simulink model "RobotRuka2012B"  (R2012b)
settings: Solver=ode45  SolverMode=SingleTasking  StartTime=0.0  StopTime=10.0  RelTol=1e-3
undefined symbols (not defined in the file): g, Kd, Kp, lc1, m0, m1, m2
libraries: fuzblock x2
settings Model: CovMetricSettings=dwe  CovHtmlReporting=off  covSaveCumulativeToWorkspaceVar=off  CovSaveSingleToWorkspaceVar=off  CovExternalEMLEnable=on  Creator=Aldin  LastModifiedBy=Aldin
settings DataIOCC: LimitDataPoints=off  SaveFormat=StructureWithTime  ReturnWorkspaceOutputs=on
settings OptimizationCC: ExpressionDepthLimit=128
settings DebuggingCC: UnderspecifiedInitializationDetection=Simplified  MergeDetectMultiDrivingBlocksExec=error  SolverPrmCheckMsg=none  FrameProcessingCompatibilityMsg=error  StateNameClashWarn=none  SFUnexpectedBacktrackingDiag=error  SFNoUnconditionalDefaultTransitionDiag=error
settings HardwareCC: ProdBitPerPointer=64  ProdLargestAtomicFloat=Float  ProdIntDivRoundTo=Zero  ProdEndianess=LittleEndian  ProdHWDeviceType=Specified
settings ModelReferenceCC: PropagateSignalLabelsOutOfModel=on
settings SFSimCC: SimUseLocalCustomCode=on
settings RTWCC: RTWUseLocalCustomCode=on
settings CodeAppCC: CustomSymbolStrType=$N$R$M_T
settings GRTTargetCC: CodeReplacementLibrary=C99 (ISO)

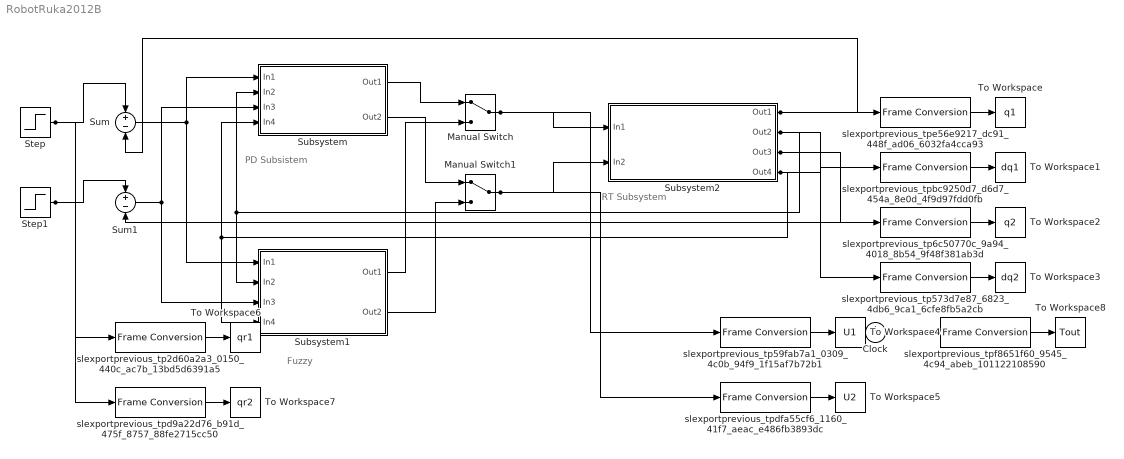
== system RobotRuka2012B ==
  note: PD Subsistem
  note: Fuzzy
  note: RT Subsystem
  Clock : Clock
  Manual Switch : ManualSwitch
  Manual Switch1 : ManualSwitch
  Step : Step  Time=0  SampleTime=0
  Step1 : Step  Time=0  SampleTime=0
  Subsystem : Subsystem
  Subsystem1 : Subsystem
  Subsystem2 : Subsystem
  Sum : Sum  Inputs=+-
  Sum1 : Sum  Inputs=+-
  To Workspace : ToWorkspace  VariableName=q1  SampleTime=-1
  To Workspace1 : ToWorkspace  VariableName=dq1  SampleTime=-1
  To Workspace2 : ToWorkspace  VariableName=q2  SampleTime=-1
  To Workspace3 : ToWorkspace  VariableName=dq2  SampleTime=-1
  To Workspace4 : ToWorkspace  VariableName=U1  SampleTime=-1
  To Workspace5 : ToWorkspace  VariableName=U2  SampleTime=-1
  To Workspace6 : ToWorkspace  VariableName=qr1  SampleTime=-1
  To Workspace7 : ToWorkspace  VariableName=qr2  SampleTime=-1
  To Workspace8 : ToWorkspace  VariableName=Tout  SampleTime=-1
  slexportprevious_tp2d60a2a3_0150_440c_ac7b_13bd5d6391a5 : FrameConversion  OutFrame=Sample-based
  slexportprevious_tp573d7e87_6823_4db6_9ca1_6cfe8fb5a2cb : FrameConversion  OutFrame=Sample-based
  slexportprevious_tp59fab7a1_0309_4c0b_94f9_1f15af7b72b1 : FrameConversion  OutFrame=Sample-based
  slexportprevious_tp6c50770c_9a94_4018_8b54_9f48f381ab3d : FrameConversion  OutFrame=Sample-based
  slexportprevious_tpbc9250d7_d6d7_454a_8e0d_4f9d97fdd0fb : FrameConversion  OutFrame=Sample-based
  slexportprevious_tpd9a22d76_b91d_475f_8757_88fe2715cc50 : FrameConversion  OutFrame=Sample-based
  slexportprevious_tpdfa55cf6_1160_41f7_aeac_e486fb3893dc : FrameConversion  OutFrame=Sample-based
  slexportprevious_tpe56e9217_dc91_448f_ad06_6032fa4cca93 : FrameConversion  OutFrame=Sample-based
  slexportprevious_tpf8651f60_9545_4c94_abeb_101122108590 : FrameConversion  OutFrame=Sample-based
  wires:
  Subsystem2/4(Out4) -> Subsystem/4(In4), Subsystem1/4(In4), slexportprevious_tp573d7e87_6823_4db6_9ca1_6cfe8fb5a2cb/1
  Subsystem1/2(Out2) -> Manual Switch1/2
  Manual Switch/1 -> Subsystem2/1(In1), slexportprevious_tp59fab7a1_0309_4c0b_94f9_1f15af7b72b1/1
  Subsystem2/1(Out1) -> Sum/2, slexportprevious_tpe56e9217_dc91_448f_ad06_6032fa4cca93/1
  Subsystem1/1(Out1) -> Manual Switch/2
  Subsystem2/3(Out3) -> Sum1/2, slexportprevious_tp6c50770c_9a94_4018_8b54_9f48f381ab3d/1
  Manual Switch1/1 -> Subsystem2/2(In2), slexportprevious_tpdfa55cf6_1160_41f7_aeac_e486fb3893dc/1
  Sum1/1 -> Subsystem1/3(In3), Subsystem/3(In3)
  Subsystem2/2(Out2) -> Subsystem1/2(In2), Subsystem/2(In2), slexportprevious_tpbc9250d7_d6d7_454a_8e0d_4f9d97fdd0fb/1
  Step1/1 -> Sum1/1, slexportprevious_tpd9a22d76_b91d_475f_8757_88fe2715cc50/1
  Sum/1 -> Subsystem/1(In1), Subsystem1/1(In1)
  Subsystem/1(Out1) -> Manual Switch/1
  Step/1 -> Sum/1, slexportprevious_tp2d60a2a3_0150_440c_ac7b_13bd5d6391a5/1
  Subsystem/2(Out2) -> Manual Switch1/1
  slexportprevious_tpe56e9217_dc91_448f_ad06_6032fa4cca93/1 -> To Workspace/1
  slexportprevious_tpbc9250d7_d6d7_454a_8e0d_4f9d97fdd0fb/1 -> To Workspace1/1
  slexportprevious_tp6c50770c_9a94_4018_8b54_9f48f381ab3d/1 -> To Workspace2/1
  slexportprevious_tp573d7e87_6823_4db6_9ca1_6cfe8fb5a2cb/1 -> To Workspace3/1
  slexportprevious_tp59fab7a1_0309_4c0b_94f9_1f15af7b72b1/1 -> To Workspace4/1
  slexportprevious_tpdfa55cf6_1160_41f7_aeac_e486fb3893dc/1 -> To Workspace5/1
  slexportprevious_tp2d60a2a3_0150_440c_ac7b_13bd5d6391a5/1 -> To Workspace6/1
  slexportprevious_tpd9a22d76_b91d_475f_8757_88fe2715cc50/1 -> To Workspace7/1
  Clock/1 -> slexportprevious_tpf8651f60_9545_4c94_abeb_101122108590/1
  slexportprevious_tpf8651f60_9545_4c94_abeb_101122108590/1 -> To Workspace8/1

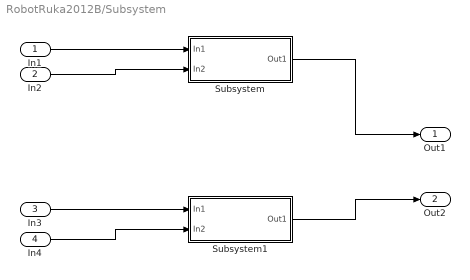
== system RobotRuka2012B/Subsystem ==
  In1 : Inport
  In2 : Inport  Port=2
  In3 : Inport  Port=3
  In4 : Inport  Port=4
  Subsystem : Subsystem
  Subsystem1 : Subsystem
  Out1 : Outport
  Out2 : Outport  Port=2
  wires:
  Subsystem/1(Out1) -> Out1/1
  In1/1 -> Subsystem/1(In1)
  In2/1 -> Subsystem/2(In2)
  In3/1 -> Subsystem1/1(In1)
  In4/1 -> Subsystem1/2(In2)
  Subsystem1/1(Out1) -> Out2/1

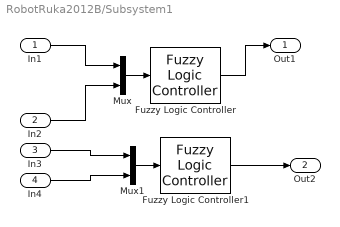
== system RobotRuka2012B/Subsystem1 ==
  In1 : Inport
  In2 : Inport  Port=2
  In3 : Inport  Port=3
  In4 : Inport  Port=4
  Fuzzy Logic Controller : fuzblock/Fuzzy Logic  Controller  FIS=rtfuzzy
  Fuzzy Logic Controller1 : fuzblock/Fuzzy Logic  Controller  FIS=rtfuzzy
  Mux : Mux  Inputs=2
  Mux1 : Mux  Inputs=2
  Out1 : Outport
  Out2 : Outport  Port=2
  wires:
  Mux/1 -> Fuzzy Logic Controller/1
  In1/1 -> Mux/1
  In2/1 -> Mux/2
  Fuzzy Logic Controller/1 -> Out1/1
  Mux1/1 -> Fuzzy Logic Controller1/1
  In3/1 -> Mux1/1
  In4/1 -> Mux1/2
  Fuzzy Logic Controller1/1 -> Out2/1

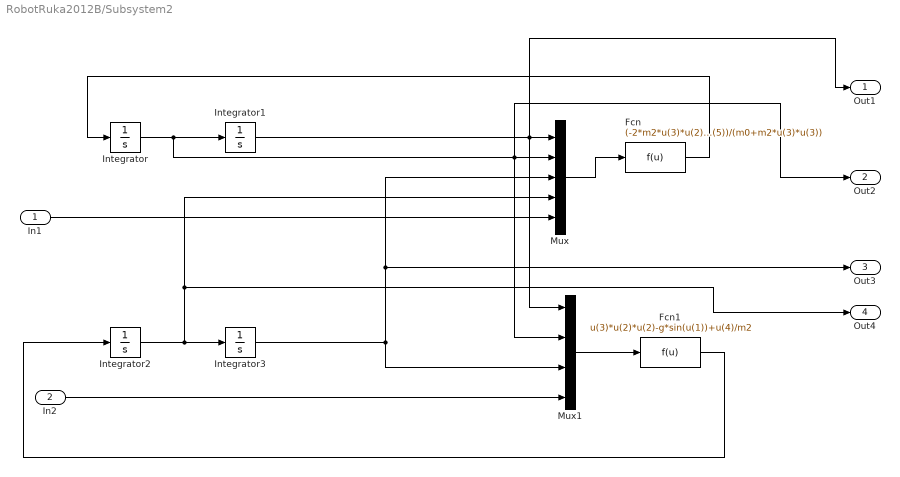
== system RobotRuka2012B/Subsystem2 ==
  In1 : Inport
  In2 : Inport  Port=2
  Fcn : Fcn  Expr=(-2*m2*u(3)*u(2)*u(4)-m1*lc1*g*cos(u(1))-m2*g*u(3)*cos(u(1))+u(5))/(m0+m2*u(3)*u(3))
  Fcn1 : Fcn  Expr=u(3)*u(2)*u(2)-g*sin(u(1))+u(4)/m2
  Integrator{,1..3} (4 alike) : Integrator
  Mux : Mux  Inputs=5
  Mux1 : Mux
  Out1 : Outport
  Out2 : Outport  Port=2
  Out3 : Outport  Port=3
  Out4 : Outport  Port=4
  wires:
  In1/1 -> Mux/5
  Mux/1 -> Fcn/1
  Fcn/1 -> Integrator/1
  Integrator/1 -> Mux1/2, Out2/1, Mux/2, Integrator1/1
  Integrator1/1 -> Mux1/1, Out1/1, Mux/1
  Fcn1/1 -> Integrator2/1
  Integrator2/1 -> Out4/1, Mux/4, Integrator3/1
  Integrator3/1 -> Out3/1, Mux/3, Mux1/3
  In2/1 -> Mux1/4
  Mux1/1 -> Fcn1/1

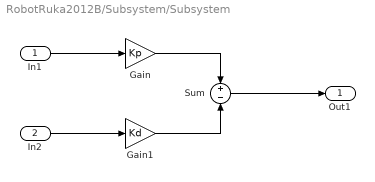
== system RobotRuka2012B/Subsystem/Subsystem ==
  In1 : Inport
  In2 : Inport  Port=2
  Gain : Gain  Gain=Kp
  Gain1 : Gain  Gain=Kd
  Sum : Sum  Inputs=+-
  Out1 : Outport
  wires:
  Gain/1 -> Sum/1
  Gain1/1 -> Sum/2
  Sum/1 -> Out1/1
  In2/1 -> Gain1/1
  In1/1 -> Gain/1

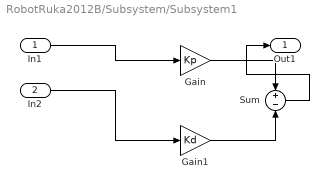
== system RobotRuka2012B/Subsystem/Subsystem1 ==
  In1 : Inport
  In2 : Inport  Port=2
  Gain : Gain  Gain=Kp
  Gain1 : Gain  Gain=Kd
  Sum : Sum  Inputs=+-
  Out1 : Outport
  wires:
  Gain1/1 -> Sum/2
  Gain/1 -> Sum/1
  In1/1 -> Gain/1
  Sum/1 -> Out1/1
  In2/1 -> Gain1/1
